simulink model "Stryfe_Simulation_2"  (R2020b)
settings: Solver=VariableStepAuto  StartTime=0.0  StopTime=10.0  RelTol=1e-3
values from neighbouring files (symbols this model uses):
  F15_TC = [0 0.25 0.5 0.75 1 1.25 1.5 2 2.25 2.5 3 3.25 ... (26 elements, 13x2)]    [F15_TC.mat]
libraries: simulink_extras x3, simulink x2, shared3dof x1, pid_lib x1
settings Model: Creator=bowen  LastModifiedBy=bowen

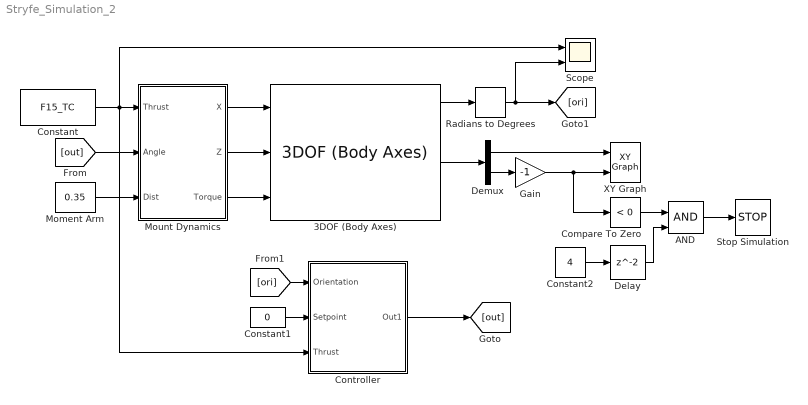
== system Stryfe_Simulation_2 ==
  3DOF (Body Axes) : shared3dof/3DOF (Body Axes)  units=Metric (MKS)  mtype=Fixed  v_ini=100  theta_ini=0  alpha_ini=0  pos_ini=[0 0]  q_ini=0  mass=1.0  mass_e=0.5  mass_f=3.0  Iyy=1.0  Iyy_e=0.5  Iyy_f=3.0  g_in=Internal  g=9.81  vre_flag=on  abi_flag=off  aMode=0  vel_statename=''  theta_statename=''  pos_statename=''  q_statename=''  mass_statename=''
      settings: SourceProductBaseCode=AE,PW,MT,UV,VE,VP
  AND : Logic  IconShape=distinctive  AllPortsSameDT=off  OutDataTypeStr=boolean
  Compare To Zero : simulink/Logic and Bit Operations/Compare To Zero  relop=<  OutDataTypeStr=boolean
  Constant : Constant  Value=F15_TC
  Constant1 : Constant  Value=0
  Constant2 : Constant  Value=4
  Controller : Subsystem
  Delay : Delay
  Demux : Demux  Outputs=2
  Gain : Gain  Gain=-1
  Moment Arm : Constant  Value=0.35
  Mount Dynamics : Subsystem
  Radians to Degrees : simulink_extras/Transformations/Radians to Degrees
  Scope : Scope  NumInputPorts=2
  Stop Simulation : Stop
  XY Graph : simulink/Sinks/XY Graph  xmin=-1  xmax=1  ymin=-1  ymax=1  st=-1
  wires:
  Constant/1 -> Scope/1, Controller/3(Thrust), Mount Dynamics/1(Thrust)
  Mount Dynamics/1(X) -> 3DOF (Body Axes)/1
  Mount Dynamics/3(Torque) -> 3DOF (Body Axes)/3
  Mount Dynamics/2(Z) -> 3DOF (Body Axes)/2
  Moment Arm/1 -> Mount Dynamics/3(Dist)
  [out] -> Mount Dynamics/2(Angle)
  Controller/1(Out1) -> [out]
  [ori] -> Controller/1(Orientation)
  Constant1/1 -> Controller/2(Setpoint)
  3DOF (Body Axes)/1 -> Radians to Degrees/1
  Radians to Degrees/1 -> Scope/2, [ori]
  3DOF (Body Axes)/4 -> Demux/1
  Demux/2 -> Gain/1
  Demux/1 -> XY Graph/1
  Gain/1 -> Compare To Zero/1, XY Graph/2
  AND/1 -> Stop Simulation/1
  Compare To Zero/1 -> AND/1
  Delay/1 -> AND/2
  Constant2/1 -> Delay/1

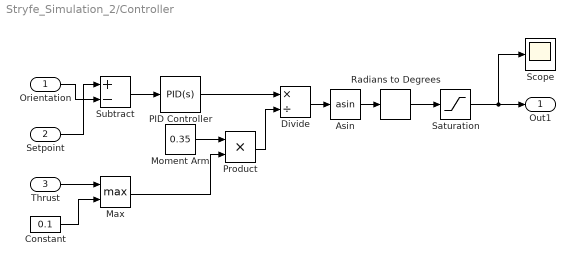
== system Stryfe_Simulation_2/Controller ==
  Orientation : Inport
  Setpoint : Inport  Port=2
  Thrust : Inport  Port=3
  Asin : Trigonometry  Operator=asin
  Constant : Constant  Value=0.1
  Divide : Product  Inputs=*/
  Max : MinMax  Function=max  Inputs=2
  Moment Arm : Constant  Value=0.35
  PID Controller : pid_lib/PID Controller  Controller=PID  Form=Parallel  TimeDomain=Continuous-time  UseExternalTs=off  SampleTime=-1  IntegratorMethod=Forward Euler  FilterMethod=Forward Euler  ControllerParametersSource=internal  P=1  I=1  D=0  UseFilter=on  N=100  TunerSelectOption=Transfer Function Based (PID Tuner App)  InitialConditionSource=internal  InitialConditionForIntegrator=0  InitialConditionForFilter=0  DifferentiatorICPrevScaledInput=0  ExternalReset=none  TrackingMode=off  Kt=1  LimitOutput=off  SatLimitsSource=internal  UpperSaturationLimit=inf  LowerSaturationLimit=-inf  LinearizeAsGain=on  AntiWindupMode=none  Kb=1  POutMin=[]  POutMax=[]  IOutMin=[]  IOutMax=[]  DOutMin=[]  DOutMax=[]  NOutMin=[]  NOutMax=[]  SumOutMin=[]  SumOutMax=[]  SaturationOutMin=[]  SaturationOutMax=[]  PParamMin=[]  PParamMax=[]  IParamMin=[]  IParamMax=[]  DParamMin=[]  DParamMax=[]  NParamMin=[]  NParamMax=[]  KbParamMin=[]  KbParamMax=[]  KtParamMin=[]  KtParamMax=[]  KbOutMin=[]  KbOutMax=[]  KtOutMin=[]  KtOutMax=[]  IntegratorOutMin=[]  IntegratorOutMax=[]  FilterOutMin=[]  FilterOutMax=[]  SumI1OutMin=[]  SumI1OutMax=[]  SumI2OutMin=[]  SumI2OutMax=[]  SumI3OutMin=[]  SumI3OutMax=[]  SumI4OutMin=[]  SumI4OutMax=[]  SumDOutMin=[]  SumDOutMax=[]  DifferentiatorOutMin=[]  DifferentiatorOutMax=[]  FilterDiffOutCoefMin=[]  FilterDiffOutCoefMax=[]  ReciprocalOutMin=[]  ReciprocalOutMax=[]  SumDenOutMin=[]  SumDenOutMax=[]  SumNumOutMin=[]  SumNumOutMax=[]  DivideOutMin=[]  DivideOutMax=[]  UdiffTsProdOutMin=[]  UdiffTsProdOutMax=[]  NTsProdOutMin=[]  NTsProdOutMax=[]  UintegralTsProdOutMin=[]  UintegralTsProdOutMax=[]  UngainTsProdOutMin=[]  UngainTsProdOutMax=[]  IntegratorContinuousStateAttributes=''  IntegratorStateMustResolveToSignalObject=off  IntegratorRTWStateStorageClass=Auto  FilterContinuousStateAttributes=''  FilterStateMustResolveToSignalObject=off  FilterRTWStateStorageClass=Auto  ParallelPVariant=InternalParameters  IdealPVariant=Disabled  IVariant=InternalParameters  DVariant=InternalParameters  IntegratorVariant=Continuous  SatVariant=Disabled  AWVariant=Passthrough  PCopyVariant=Disabled  TRVariant=Disabled  FdbkBlocksVariant=Forward  IdealPFdbkVariant=Disabled  SatFdbkVariant=Disabled  DerivativeFilterVariant=ContFilter  NVariant=InternalParameters  NCopyVariant=Disabled  FilterICVariant=InternalICsFilter  IntegratorICVariant=InternalICs  ExternalResetVariant=Disabled  TRSumVariant=Passthrough  SumFdbkVariant=Disabled  SumVariant=Sum_PID  TsampFilterVariant=InternalTs  TsampNgainVariant=Passthrough  TsampIntegralVariant=Passthrough  ExternalSaturationOutDataTypeStr=Inherit: Same as second input
  Product : Product
  Radians to Degrees : simulink_extras/Transformations/Radians to Degrees
  Saturation : Saturate  UpperLimit=5  LowerLimit=-5
  Scope : Scope
  Subtract : Sum  Inputs=+-
  Out1 : Outport
  wires:
  Setpoint/1 -> Subtract/1
  Orientation/1 -> Subtract/2
  Subtract/1 -> PID Controller/1
  PID Controller/1 -> Divide/1
  Divide/1 -> Asin/1
  Asin/1 -> Radians to Degrees/1
  Thrust/1 -> Max/1
  Constant/1 -> Max/2
  Moment Arm/1 -> Product/1
  Product/1 -> Divide/2
  Radians to Degrees/1 -> Saturation/1
  Saturation/1 -> Scope/1, Out1/1
  Max/1 -> Product/2

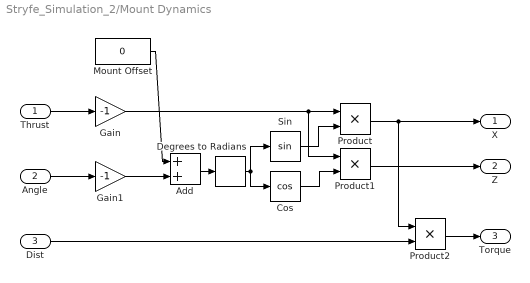
== system Stryfe_Simulation_2/Mount Dynamics ==
  Thrust : Inport
  Angle : Inport  Port=2
  Dist : Inport  Port=3
  Add : Sum
  Cos : Trigonometry  Operator=cos
  Degrees to Radians : simulink_extras/Transformations/Degrees to Radians
  Gain : Gain  Gain=-1
  Gain1 : Gain  Gain=-1
  Mount Offset : Constant  Value=0
  Product : Product
  Product1 : Product
  Product2 : Product
  Sin : Trigonometry
  X : Outport
  Z : Outport  Port=2
  Torque : Outport  Port=3
  wires:
  Gain1/1 -> Add/2
  Mount Offset/1 -> Add/1
  Add/1 -> Degrees to Radians/1
  Degrees to Radians/1 -> Cos/1, Sin/1
  Cos/1 -> Product1/2
  Sin/1 -> Product/2
  Gain/1 -> Product1/1, Product/1
  Thrust/1 -> Gain/1
  Product/1 -> Product2/1, X/1
  Product2/1 -> Torque/1
  Dist/1 -> Product2/2
  Angle/1 -> Gain1/1
  Product1/1 -> Z/1
